simulink library "TYPEC_MASTER"  (Simulink 8.8)
settings: Solver=ode45  StartTime=0.0  StopTime=10.0  RelTol=1e-3  EnableMultiTasking=on
libraries: cdsEpicsOut x60, cdsFilt x45, cdsTP x20, cdsEpicsIn x18, cdsFiltCtrl x18, VIS_LIB x16, cdsMuxMatrix x8, cdsEpicsStringIn x6, cdsEpicsBinIn x4, lockin x4, cdsFunctionCall x4, STATE_BIO_MASTER x2
(part 1 of 7)
settings Model: SuppressorTable=22 serialization::archive 11 0 3 0 0 0 11 0  Creator=controls  LastModifiedBy=controls

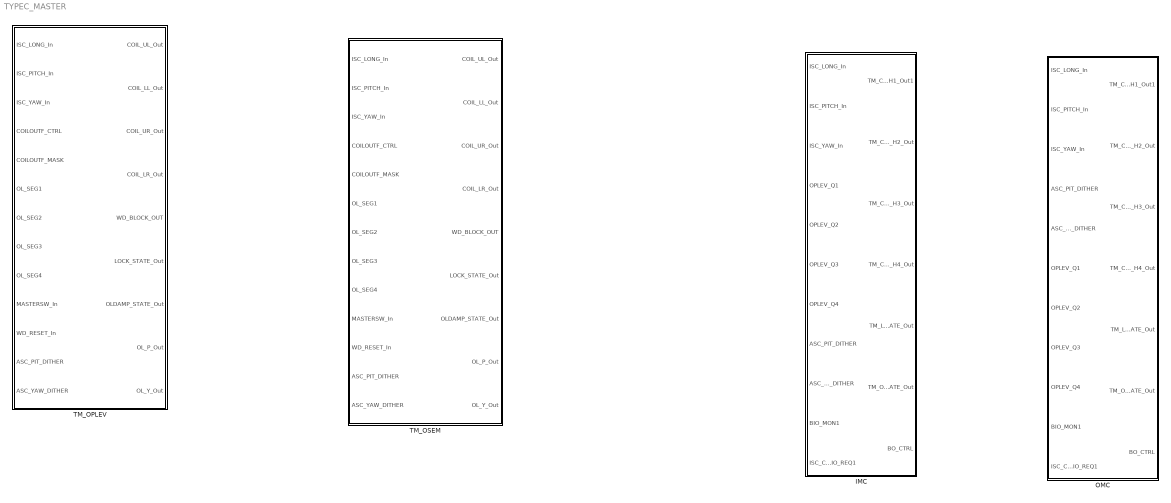
== system TYPEC_MASTER ==
  IMC : Subsystem  Description=TYPEC SINGLE MASTER
      settings: AttributesFormatString=%<Description>
  OMC : Subsystem  Description=TYPEC SINGLE MASTER
      settings: AttributesFormatString=%<Description>
  TM_OPLEV : Subsystem
  TM_OSEM : Subsystem

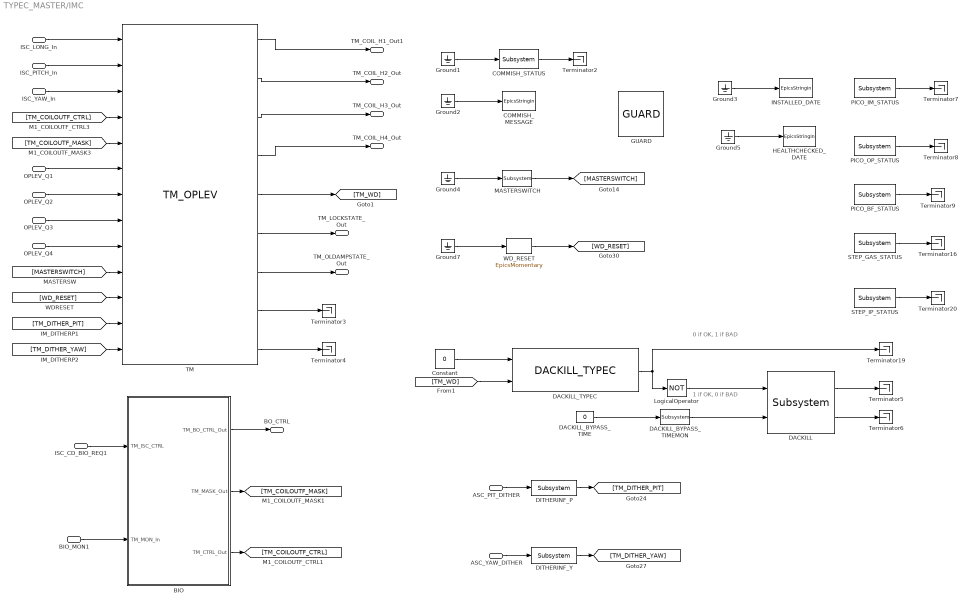
== system TYPEC_MASTER/IMC ==
  note: 0 if OK, 1 if BAD
  note: 1 if OK, 0 if BAD
  ISC_LONG_In : Inport
  ISC_PITCH_In : Inport  Port=2
  ISC_YAW_In : Inport  Port=3
  OPLEV_Q1 : Inport  Port=4
  OPLEV_Q2 : Inport  Port=5
  OPLEV_Q3 : Inport  Port=6
  OPLEV_Q4 : Inport  Port=7
  ASC_PIT_DITHER : Inport  Port=8
  ASC_YAW_DITHER : Inport  Port=9
  BIO_MON1 : Inport  Port=10
  ISC_CD_BIO_REQ1 : Inport  Port=11
  BIO : Subsystem
  COMMISH_MESSAGE : cdsEpicsStringIn/EpicsStringIn  Tag=cdsEpicsStringIn  Description=cdsEpicsStringIn
      settings: AttributesFormatString=%<Tag>
  COMMISH_STATUS : cdsEpicsBinIn/Subsystem  Tag=cdsEpicsBinIn  Description=|
      | Purpose:                                                                            
      | Create an EPICS binary (0 or 1) input channel to the FE realtime controls.          
      |                                                                                     
      | Operation:                                                                          
      | Outputs value from an EPICS ai record. Value is binary input (bi Epics record type).
      |                                                                                     
      | Usage:                                                                              
      | Name the part with the desired EPICS channel name.
      settings: AttributesFormatString=%<Tag>
  Constant : Constant  Value=0
  DACKILL : cdsDacKill/Subsystem  Description=cdsDacKill
      settings: AttributesFormatString=%<Description>
  DACKILL_BYPASS_TIME : Constant  Value=0
  DACKILL_BYPASS_TIMEMON : cdsEpicsOut/Subsystem  Tag=cdsEpicsOutput  Description=|
      | Purpose:                                          
      | Output a FE signal to an EPICS channel.           
      |                                                   
      | Operation:                                        
      | Takes input value and passes it to EPICS record.  
      |                                                   
      | Usage:                                            
      | Name the part with the desired EPICS rrecord name.
      settings: AttributesFormatString=%<Tag>
  DACKILL_TYPEC : VIS_LIB/DACKILL_TYPEC 
  DITHERINF_P : cdsFilt/Subsystem  Tag=cdsFilt  Description=|
      | Purpose:                                                                                                                                                                                                                                  
      | Standard CDS IIR filter module.                                                                                                                                                                                                           
      |                                                                                                                                                                                                                                           
      | Operation:                                                                                                                                                                                                                                
      | Consists of 10 second order section IIR filters, plus a ramped gain stage. In FE code, also provides pre-defined test points and excitation channel inputs. The filter coefficients are defined in the LIGO system using the 'foton' tool.
      |                                                                                                                                                                                                                                           
      | Usage:                                                                                                                                                                                                                                    
      | Name the part with the desired filter module name.
      settings: AttributesFormatString=%<Tag>
  DITHERINF_Y : cdsFilt/Subsystem  Tag=cdsFilt  Description=|
      | Purpose:                                                                                                                                                                                                                                  
      | Standard CDS IIR filter module.                                                                                                                                                                                                           
      |                                                                                                                                                                                                                                           
      | Operation:                                                                                                                                                                                                                                
      | Consists of 10 second order section IIR filters, plus a ramped gain stage. In FE code, also provides pre-defined test points and excitation channel inputs. The filter coefficients are defined in the LIGO system using the 'foton' tool.
      |                                                                                                                                                                                                                                           
      | Usage:                                                                                                                                                                                                                                    
      | Name the part with the desired filter module name.
      settings: AttributesFormatString=%<Tag>
  GUARD : ISC_common/GUARD
  Ground{1..5,7} (6 alike) : Ground
  HEALTHCHECKED_DATE : cdsEpicsStringIn/EpicsStringIn  Tag=cdsEpicsStringIn  Description=cdsEpicsStringIn
      settings: AttributesFormatString=%<Tag>
  INSTALLED_DATE : cdsEpicsStringIn/EpicsStringIn  Tag=cdsEpicsStringIn  Description=cdsEpicsStringIn
      settings: AttributesFormatString=%<Tag>
  LogicalOperator : Logic  Operator=NOT  AllPortsSameDT=off  OutDataTypeStr=boolean
  MASTERSWITCH : cdsEpicsBinIn/Subsystem  Tag=cdsEpicsBinIn  Description=|
      | Purpose:                                                                            
      | Create an EPICS binary (0 or 1) input channel to the FE realtime controls.          
      |                                                                                     
      | Operation:                                                                          
      | Outputs value from an EPICS ai record. Value is binary input (bi Epics record type).
      |                                                                                     
      | Usage:                                                                              
      | Name the part with the desired EPICS channel name.
      settings: AttributesFormatString=%<Tag>
  PICO_BF_STATUS : cdsEpicsIn/Subsystem  Tag=cdsEpicsIn  Description=|
      | Purpose:                                                                              
      | Create an EPICS input channel connection to the FE realtime controls.                 
      |                                                                                       
      | Operation:                                                                            
      | Outputs value from an EPICS ai record. Value is floating point with a precision of 3..
      |                                                                                       
      | Usage:                                                                                
      | Name the part with the desired EPICS channel name.
      settings: AttributesFormatString=%<Tag>
  PICO_IM_STATUS : cdsEpicsIn/Subsystem  Tag=cdsEpicsIn  Description=|
      | Purpose:                                                                              
      | Create an EPICS input channel connection to the FE realtime controls.                 
      |                                                                                       
      | Operation:                                                                            
      | Outputs value from an EPICS ai record. Value is floating point with a precision of 3..
      |                                                                                       
      | Usage:                                                                                
      | Name the part with the desired EPICS channel name.
      settings: AttributesFormatString=%<Tag>
  PICO_OP_STATUS : cdsEpicsIn/Subsystem  Tag=cdsEpicsIn  Description=|
      | Purpose:                                                                              
      | Create an EPICS input channel connection to the FE realtime controls.                 
      |                                                                                       
      | Operation:                                                                            
      | Outputs value from an EPICS ai record. Value is floating point with a precision of 3..
      |                                                                                       
      | Usage:                                                                                
      | Name the part with the desired EPICS channel name.
      settings: AttributesFormatString=%<Tag>
  STEP_GAS_STATUS : cdsEpicsIn/Subsystem  Tag=cdsEpicsIn  Description=|
      | Purpose:                                                                              
      | Create an EPICS input channel connection to the FE realtime controls.                 
      |                                                                                       
      | Operation:                                                                            
      | Outputs value from an EPICS ai record. Value is floating point with a precision of 3..
      |                                                                                       
      | Usage:                                                                                
      | Name the part with the desired EPICS channel name.
      settings: AttributesFormatString=%<Tag>
  STEP_IP_STATUS : cdsEpicsIn/Subsystem  Tag=cdsEpicsIn  Description=|
      | Purpose:                                                                              
      | Create an EPICS input channel connection to the FE realtime controls.                 
      |                                                                                       
      | Operation:                                                                            
      | Outputs value from an EPICS ai record. Value is floating point with a precision of 3..
      |                                                                                       
      | Usage:                                                                                
      | Name the part with the desired EPICS channel name.
      settings: AttributesFormatString=%<Tag>
  TM : TYPEC_MASTER/TM_OPLEV
  Terminator{2..9,16,19..20} (11 alike) : Terminator
  WD_RESET : cdsEpicsMomentary/EpicsMomentary  Tag=cdsEpicsMomentary
      settings: AttributesFormatString=%<Tag>
  TM_COIL_H1_Out1 : Outport
  TM_COIL_H2_Out : Outport  Port=2
  TM_COIL_H3_Out : Outport  Port=3
  TM_COIL_H4_Out : Outport  Port=4
  TM_LOCKSTATE_Out : Outport  Port=5
  TM_OLDAMPSTATE_Out : Outport  Port=6
  BO_CTRL : Outport  Port=7
  wires:
  TM/9 -> Terminator4/1
  TM/2 -> TM_COIL_H2_Out/1
  TM/1 -> TM_COIL_H1_Out1/1
  TM/4 -> TM_COIL_H4_Out/1
  TM/3 -> TM_COIL_H3_Out/1
  [TM_WD] -> DACKILL_TYPEC/2
  Constant/1 -> DACKILL_TYPEC/1
  DACKILL_TYPEC/1 -> Terminator19/1, LogicalOperator/1
  LogicalOperator/1 -> DACKILL/1
  DACKILL_BYPASS_TIMEMON/1 -> DACKILL/2
  DACKILL_BYPASS_TIME/1 -> DACKILL_BYPASS_TIMEMON/1
  DACKILL/1 -> Terminator5/1
  DACKILL/2 -> Terminator6/1
  [TM_DITHER_YAW] -> TM/13
  [TM_DITHER_PIT] -> TM/12
  DITHERINF_Y/1 -> [TM_DITHER_YAW]
  DITHERINF_P/1 -> [TM_DITHER_PIT]
  ASC_PIT_DITHER/1 -> DITHERINF_P/1
  ASC_YAW_DITHER/1 -> DITHERINF_Y/1
  Ground1/1 -> COMMISH_STATUS/1
  COMMISH_STATUS/1 -> Terminator2/1
  Ground2/1 -> COMMISH_MESSAGE/1
  ISC_LONG_In/1 -> TM/1
  TM/5 -> [TM_WD]
  MASTERSWITCH/1 -> [MASTERSWITCH]
  Ground4/1 -> MASTERSWITCH/1
  OPLEV_Q1/1 -> TM/6
  OPLEV_Q2/1 -> TM/7
  OPLEV_Q3/1 -> TM/8
  ISC_PITCH_In/1 -> TM/2
  ISC_YAW_In/1 -> TM/3
  OPLEV_Q4/1 -> TM/9
  [MASTERSWITCH] -> TM/10
  Ground7/1 -> WD_RESET/1
  WD_RESET/1 -> [WD_RESET]
  [WD_RESET] -> TM/11
  BIO_MON1/1 -> BIO/2(TM_MON_In)
  ISC_CD_BIO_REQ1/1 -> BIO/1(TM_ISC_CTRL)
  BIO/2(TM_MASK_Out) -> [TM_COILOUTF_MASK]
  BIO/3(TM_CTRL_Out) -> [TM_COILOUTF_CTRL]
  [TM_COILOUTF_CTRL] -> TM/4
  [TM_COILOUTF_MASK] -> TM/5
  BIO/1(TM_BO_CTRL_Out) -> BO_CTRL/1
  TM/6 -> TM_LOCKSTATE_Out/1
  TM/7 -> TM_OLDAMPSTATE_Out/1
  TM/8 -> Terminator3/1
  Ground3/1 -> INSTALLED_DATE/1
  Ground5/1 -> HEALTHCHECKED_DATE/1
  STEP_IP_STATUS/1 -> Terminator20/1
  STEP_GAS_STATUS/1 -> Terminator16/1
  PICO_BF_STATUS/1 -> Terminator9/1
  PICO_IM_STATUS/1 -> Terminator7/1
  PICO_OP_STATUS/1 -> Terminator8/1

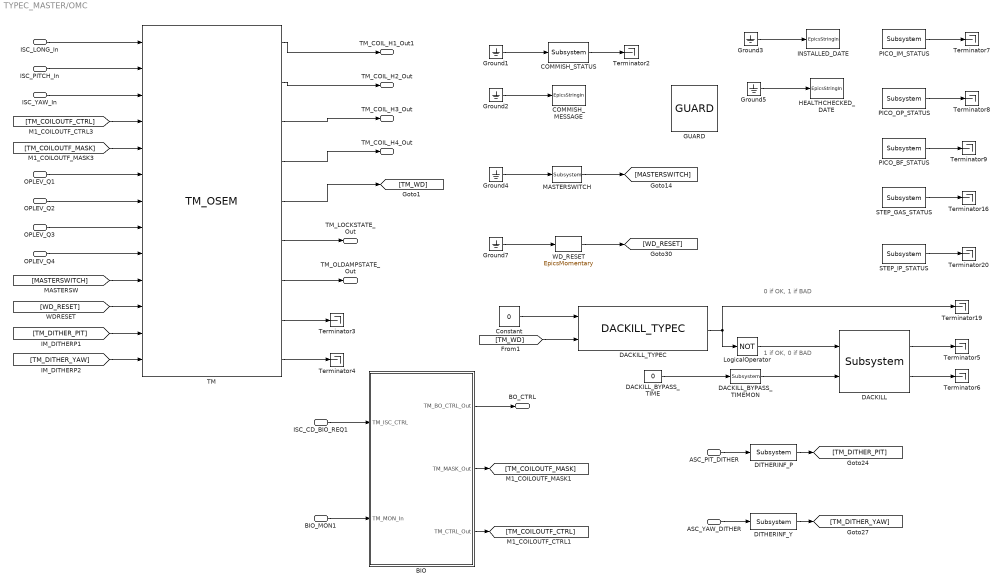
== system TYPEC_MASTER/OMC ==
  note: 0 if OK, 1 if BAD
  note: 1 if OK, 0 if BAD
  ISC_LONG_In : Inport
  ISC_PITCH_In : Inport  Port=2
  ISC_YAW_In : Inport  Port=3
  ASC_PIT_DITHER : Inport  Port=4
  ASC_YAW_DITHER : Inport  Port=5
  OPLEV_Q1 : Inport  Port=6
  OPLEV_Q2 : Inport  Port=7
  OPLEV_Q3 : Inport  Port=8
  OPLEV_Q4 : Inport  Port=9
  BIO_MON1 : Inport  Port=10
  ISC_CD_BIO_REQ1 : Inport  Port=11
  BIO : Subsystem
  COMMISH_MESSAGE : cdsEpicsStringIn/EpicsStringIn  Tag=cdsEpicsStringIn  Description=cdsEpicsStringIn
      settings: AttributesFormatString=%<Tag>
  COMMISH_STATUS : cdsEpicsBinIn/Subsystem  Tag=cdsEpicsBinIn  Description=|
      | Purpose:                                                                            
      | Create an EPICS binary (0 or 1) input channel to the FE realtime controls.          
      |                                                                                     
      | Operation:                                                                          
      | Outputs value from an EPICS ai record. Value is binary input (bi Epics record type).
      |                                                                                     
      | Usage:                                                                              
      | Name the part with the desired EPICS channel name.
      settings: AttributesFormatString=%<Tag>
  Constant : Constant  Value=0
  DACKILL : cdsDacKill/Subsystem  Description=cdsDacKill
      settings: AttributesFormatString=%<Description>
  DACKILL_BYPASS_TIME : Constant  Value=0
  DACKILL_BYPASS_TIMEMON : cdsEpicsOut/Subsystem  Tag=cdsEpicsOutput  Description=|
      | Purpose:                                          
      | Output a FE signal to an EPICS channel.           
      |                                                   
      | Operation:                                        
      | Takes input value and passes it to EPICS record.  
      |                                                   
      | Usage:                                            
      | Name the part with the desired EPICS rrecord name.
      settings: AttributesFormatString=%<Tag>
  DACKILL_TYPEC : VIS_LIB/DACKILL_TYPEC 
  DITHERINF_P : cdsFilt/Subsystem  Tag=cdsFilt  Description=|
      | Purpose:                                                                                                                                                                                                                                  
      | Standard CDS IIR filter module.                                                                                                                                                                                                           
      |                                                                                                                                                                                                                                           
      | Operation:                                                                                                                                                                                                                                
      | Consists of 10 second order section IIR filters, plus a ramped gain stage. In FE code, also provides pre-defined test points and excitation channel inputs. The filter coefficients are defined in the LIGO system using the 'foton' tool.
      |                                                                                                                                                                                                                                           
      | Usage:                                                                                                                                                                                                                                    
      | Name the part with the desired filter module name.
      settings: AttributesFormatString=%<Tag>
  DITHERINF_Y : cdsFilt/Subsystem  Tag=cdsFilt  Description=|
      | Purpose:                                                                                                                                                                                                                                  
      | Standard CDS IIR filter module.                                                                                                                                                                                                           
      |                                                                                                                                                                                                                                           
      | Operation:                                                                                                                                                                                                                                
      | Consists of 10 second order section IIR filters, plus a ramped gain stage. In FE code, also provides pre-defined test points and excitation channel inputs. The filter coefficients are defined in the LIGO system using the 'foton' tool.
      |                                                                                                                                                                                                                                           
      | Usage:                                                                                                                                                                                                                                    
      | Name the part with the desired filter module name.
      settings: AttributesFormatString=%<Tag>
  GUARD : ISC_common/GUARD
  Ground{1..5,7} (6 alike) : Ground
  HEALTHCHECKED_DATE : cdsEpicsStringIn/EpicsStringIn  Tag=cdsEpicsStringIn  Description=cdsEpicsStringIn
      settings: AttributesFormatString=%<Tag>
  INSTALLED_DATE : cdsEpicsStringIn/EpicsStringIn  Tag=cdsEpicsStringIn  Description=cdsEpicsStringIn
      settings: AttributesFormatString=%<Tag>
  LogicalOperator : Logic  Operator=NOT  AllPortsSameDT=off  OutDataTypeStr=boolean
  MASTERSWITCH : cdsEpicsBinIn/Subsystem  Tag=cdsEpicsBinIn  Description=|
      | Purpose:                                                                            
      | Create an EPICS binary (0 or 1) input channel to the FE realtime controls.          
      |                                                                                     
      | Operation:                                                                          
      | Outputs value from an EPICS ai record. Value is binary input (bi Epics record type).
      |                                                                                     
      | Usage:                                                                              
      | Name the part with the desired EPICS channel name.
      settings: AttributesFormatString=%<Tag>
  PICO_BF_STATUS : cdsEpicsIn/Subsystem  Tag=cdsEpicsIn  Description=|
      | Purpose:                                                                              
      | Create an EPICS input channel connection to the FE realtime controls.                 
      |                                                                                       
      | Operation:                                                                            
      | Outputs value from an EPICS ai record. Value is floating point with a precision of 3..
      |                                                                                       
      | Usage:                                                                                
      | Name the part with the desired EPICS channel name.
      settings: AttributesFormatString=%<Tag>
  PICO_IM_STATUS : cdsEpicsIn/Subsystem  Tag=cdsEpicsIn  Description=|
      | Purpose:                                                                              
      | Create an EPICS input channel connection to the FE realtime controls.                 
      |                                                                                       
      | Operation:                                                                            
      | Outputs value from an EPICS ai record. Value is floating point with a precision of 3..
      |                                                                                       
      | Usage:                                                                                
      | Name the part with the desired EPICS channel name.
      settings: AttributesFormatString=%<Tag>
  PICO_OP_STATUS : cdsEpicsIn/Subsystem  Tag=cdsEpicsIn  Description=|
      | Purpose:                                                                              
      | Create an EPICS input channel connection to the FE realtime controls.                 
      |                                                                                       
      | Operation:                                                                            
      | Outputs value from an EPICS ai record. Value is floating point with a precision of 3..
      |                                                                                       
      | Usage:                                                                                
      | Name the part with the desired EPICS channel name.
      settings: AttributesFormatString=%<Tag>
  STEP_GAS_STATUS : cdsEpicsIn/Subsystem  Tag=cdsEpicsIn  Description=|
      | Purpose:                                                                              
      | Create an EPICS input channel connection to the FE realtime controls.                 
      |                                                                                       
      | Operation:                                                                            
      | Outputs value from an EPICS ai record. Value is floating point with a precision of 3..
      |                                                                                       
      | Usage:                                                                                
      | Name the part with the desired EPICS channel name.
      settings: AttributesFormatString=%<Tag>
  STEP_IP_STATUS : cdsEpicsIn/Subsystem  Tag=cdsEpicsIn  Description=|
      | Purpose:                                                                              
      | Create an EPICS input channel connection to the FE realtime controls.                 
      |                                                                                       
      | Operation:                                                                            
      | Outputs value from an EPICS ai record. Value is floating point with a precision of 3..
      |                                                                                       
      | Usage:                                                                                
      | Name the part with the desired EPICS channel name.
      settings: AttributesFormatString=%<Tag>
  TM : TYPEC_MASTER/TM_OSEM
  Terminator{2..9,16,19..20} (11 alike) : Terminator
  WD_RESET : cdsEpicsMomentary/EpicsMomentary  Tag=cdsEpicsMomentary
      settings: AttributesFormatString=%<Tag>
  TM_COIL_H1_Out1 : Outport
  TM_COIL_H2_Out : Outport  Port=2
  TM_COIL_H3_Out : Outport  Port=3
  TM_COIL_H4_Out : Outport  Port=4
  TM_LOCKSTATE_Out : Outport  Port=5
  TM_OLDAMPSTATE_Out : Outport  Port=6
  BO_CTRL : Outport  Port=7
  wires:
  TM/9 -> Terminator4/1
  TM/2 -> TM_COIL_H2_Out/1
  TM/1 -> TM_COIL_H1_Out1/1
  TM/4 -> TM_COIL_H4_Out/1
  TM/3 -> TM_COIL_H3_Out/1
  [TM_WD] -> DACKILL_TYPEC/2
  Constant/1 -> DACKILL_TYPEC/1
  DACKILL_TYPEC/1 -> Terminator19/1, LogicalOperator/1
  LogicalOperator/1 -> DACKILL/1
  DACKILL_BYPASS_TIMEMON/1 -> DACKILL/2
  DACKILL_BYPASS_TIME/1 -> DACKILL_BYPASS_TIMEMON/1
  DACKILL/1 -> Terminator5/1
  DACKILL/2 -> Terminator6/1
  [TM_DITHER_YAW] -> TM/13
  [TM_DITHER_PIT] -> TM/12
  DITHERINF_Y/1 -> [TM_DITHER_YAW]
  DITHERINF_P/1 -> [TM_DITHER_PIT]
  ASC_PIT_DITHER/1 -> DITHERINF_P/1
  ASC_YAW_DITHER/1 -> DITHERINF_Y/1
  Ground1/1 -> COMMISH_STATUS/1
  COMMISH_STATUS/1 -> Terminator2/1
  Ground2/1 -> COMMISH_MESSAGE/1
  ISC_LONG_In/1 -> TM/1
  TM/5 -> [TM_WD]
  MASTERSWITCH/1 -> [MASTERSWITCH]
  Ground4/1 -> MASTERSWITCH/1
  OPLEV_Q1/1 -> TM/6
  OPLEV_Q2/1 -> TM/7
  OPLEV_Q3/1 -> TM/8
  ISC_PITCH_In/1 -> TM/2
  ISC_YAW_In/1 -> TM/3
  OPLEV_Q4/1 -> TM/9
  [MASTERSWITCH] -> TM/10
  Ground7/1 -> WD_RESET/1
  WD_RESET/1 -> [WD_RESET]
  [WD_RESET] -> TM/11
  BIO_MON1/1 -> BIO/2(TM_MON_In)
  ISC_CD_BIO_REQ1/1 -> BIO/1(TM_ISC_CTRL)
  BIO/2(TM_MASK_Out) -> [TM_COILOUTF_MASK]
  BIO/3(TM_CTRL_Out) -> [TM_COILOUTF_CTRL]
  [TM_COILOUTF_CTRL] -> TM/4
  [TM_COILOUTF_MASK] -> TM/5
  BIO/1(TM_BO_CTRL_Out) -> BO_CTRL/1
  TM/6 -> TM_LOCKSTATE_Out/1
  TM/7 -> TM_OLDAMPSTATE_Out/1
  TM/8 -> Terminator3/1
  Ground3/1 -> INSTALLED_DATE/1
  Ground5/1 -> HEALTHCHECKED_DATE/1
  STEP_IP_STATUS/1 -> Terminator20/1
  STEP_GAS_STATUS/1 -> Terminator16/1
  PICO_BF_STATUS/1 -> Terminator9/1
  PICO_IM_STATUS/1 -> Terminator7/1
  PICO_OP_STATUS/1 -> Terminator8/1

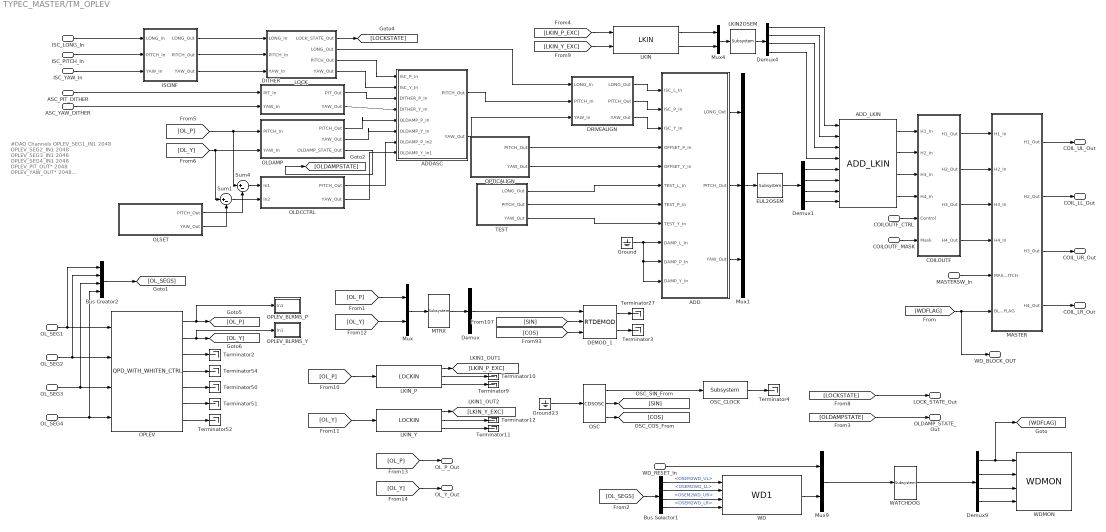
== system TYPEC_MASTER/TM_OPLEV ==
  note: #DAQ Channels
      | OPLEV_SEG1_IN1 2048
      | OPLEV_SEG2_IN1 2048
      | OPLEV_SEG3_IN1 2048
      | OPLEV_SEG4_IN1 2048
      | OPLEV_PIT_OUT* 2048
      | OPLEV_YAW_OUT* 2048
      | OPLEV_SUM_OUT 2048
      | ISCINF_L_IN1 2048
  ISC_LONG_In : Inport
  ISC_PITCH_In : Inport  Port=2
  ISC_YAW_In : Inport  Port=3
  COILOUTF_CTRL : Inport  Port=4
  COILOUTF_MASK : Inport  Port=5
  OL_SEG1 : Inport  Port=6
  OL_SEG2 : Inport  Port=7
  OL_SEG3 : Inport  Port=8
  OL_SEG4 : Inport  Port=9
  MASTERSW_In : Inport  Port=10
  WD_RESET_In : Inport  Port=11
  ASC_PIT_DITHER : Inport  Port=12
  ASC_YAW_DITHER : Inport  Port=13
  ADD : Subsystem
  ADDASC : Subsystem
  ADD_LKIN : VIS_LIB/ADD_LKIN
  Bus Creator2 : BusCreator  Inputs='OSEM2WD_UL','OSEM2WD_LL','OSEM2WD_UR','OSEM2WD_LR'
  Bus Selector1 : BusSelector  OutputSignals=OSEM2WD_UL,OSEM2WD_LL,OSEM2WD_UR,OSEM2WD_LR
  COILOUTF : Subsystem
  DEMOD_1 : VIS_LIB/RTDEMOD
  DITHER : Subsystem
  DRIVEALIGN : Subsystem
  Demux : Demux  Outputs=1
  Demux1 : Demux
  Demux4 : Demux
  Demux9 : Demux
  EUL2OSEM : cdsMuxMatrix/Subsystem  Tag=cdsMuxMatrix  Description=Any size matrix. Inputs and outputs must be connected using Mux and Demux parts.
      settings: AttributesFormatString=%<Tag>
  Ground : Ground
  Ground23 : Ground
  ISCINF : Subsystem
  LKIN : VIS_LIB/LKIN
  LKIN2OSEM : cdsMuxMatrix/Subsystem  Tag=cdsMuxMatrix  Description=Any size matrix. Inputs and outputs must be connected using Mux and Demux parts.
      settings: AttributesFormatString=%<Tag>
  LKIN_P : lockin/LOCKIN  Description=ADL=LOCKIN.adl
      settings: AttributesFormatString=%<Tag>
  LKIN_Y : lockin/LOCKIN  Description=ADL=LOCKIN.adl
      settings: AttributesFormatString=%<Tag>
  LOCK : Subsystem
  MASTER : Subsystem
  MTRX : cdsMuxMatrix/Subsystem  Tag=cdsMuxMatrix  Description=Any size matrix. Inputs and outputs must be connected using Mux and Demux parts.
      settings: AttributesFormatString=%<Tag>
  Mux : Mux  Inputs=2
  Mux1 : Mux  Inputs=3
  Mux4 : Mux  Inputs=2
  Mux9 : Mux  Inputs=2
  OLDAMP : Subsystem
  OLDCCTRL : Subsystem
  OLSET : Subsystem
  OPLEV : VIS_LIB/QPD_WITH_WHITEN_CTRL
  OPLEV_BLRMS_P : Subsystem
  OPLEV_BLRMS_Y : Subsystem
  OPTICALIGN : Subsystem
  OSC : VIS_LIB/CDSOSC  Description=ADL=OSC.adl
  OSC_CLOCK : cdsEpicsOut/Subsystem  Tag=cdsEpicsOutput  Description=|
      | Purpose:                                          
      | Output a FE signal to an EPICS channel.           
      |                                                   
      | Operation:                                        
      | Takes input value and passes it to EPICS record.  
      |                                                   
      | Usage:                                            
      | Name the part with the desired EPICS rrecord name.
      settings: AttributesFormatString=%<Tag>
  Sum1 : Sum  Inputs=|+-
  Sum4 : Sum  Inputs=|+-
  TEST : Subsystem
  Terminator{2..4,9..12,27,50..52,54} (12 alike) : Terminator
  WATCHDOG : cdsFunctionCall/Subsystem  Tag=cdsFunctionCall  Description=inline OSEMWATCHDOG /opt/rtcds/userapps/release/vis/common/src/WATCHDOG.c
      settings: AttributesFormatString=%<Tag>\n%<Description>
  WD : VIS_LIB/WD1
  WDMON : VIS_LIB/WDMON
  COIL_UL_Out : Outport
  COIL_LL_Out : Outport  Port=2
  COIL_UR_Out : Outport  Port=3
  COIL_LR_Out : Outport  Port=4
  WD_BLOCK_OUT : Outport  Port=5
  LOCK_STATE_Out : Outport  Port=6
  OLDAMP_STATE_Out : Outport  Port=7
  OL_P_Out : Outport  Port=8
  OL_Y_Out : Outport  Port=9
  wires:
  OLDCCTRL/2(YAW_Out) -> ADDASC/8(OLDAMP_Y_In1)
  OLDCCTRL/1(PITCH_Out) -> ADDASC/7(OLDAMP_P_In2)
  OLSET/2(YAW_Out) -> Sum1/2
  Sum1/1 -> OLDCCTRL/2(In2)
  Sum4/1 -> OLDCCTRL/1(In1)
  OLSET/1(PITCH_Out) -> Sum4/2
  MASTERSW_In/1 -> MASTER/5(MASTERSWITCH)
  COILOUTF/2(H2_Out) -> MASTER/2(H2_In)
  Ground/1 -> ADD/9(DAMP_L_In), ADD/11(DAMP_Y_In), ADD/10(DAMP_P_In)
  Bus Creator2/1 -> [OL_SEGS]
  [OL_Y] -> OL_Y_Out/1
  [OL_P] -> OL_P_Out/1
  [OL_Y] -> Mux/2
  [OL_P] -> Mux/1
  OSC/3 -> [COS]
  OSC/2 -> [SIN]
  OSC_CLOCK/1 -> Terminator4/1
  OSC/1 -> OSC_CLOCK/1
  Ground23/1 -> OSC/1
  DEMOD_1/2 -> Terminator3/1
  DEMOD_1/1 -> Terminator27/1
  [COS] -> DEMOD_1/3
  [SIN] -> DEMOD_1/2
  Demux/1 -> DEMOD_1/1
  MTRX/1 -> Demux/1
  Mux/1 -> MTRX/1
  ISCINF/3(YAW_Out) -> LOCK/3(YAW_In)
  ISCINF/2(PITCH_Out) -> LOCK/2(PITCH_In)
  ISCINF/1(LONG_Out) -> LOCK/1(LONG_In)
  ISC_PITCH_In/1 -> ISCINF/2(PITCH_In)
  ISC_LONG_In/1 -> ISCINF/1(LONG_In)
  ISC_YAW_In/1 -> ISCINF/3(YAW_In)
  WD/1 -> Mux9/2
  [LKIN_Y_EXC] -> LKIN/2
  [LKIN_P_EXC] -> LKIN/1
  LKIN_Y/3 -> Terminator11/1
  LKIN_Y/2 -> Terminator12/1
  [OL_Y] -> LKIN_Y/1
  LKIN_Y/1 -> [LKIN_Y_EXC]
  LKIN_P/1 -> [LKIN_P_EXC]
  LKIN_P/3 -> Terminator9/1
  LKIN_P/2 -> Terminator10/1
  [OL_P] -> LKIN_P/1
  LOCK/1(LOCK_STATE_Out) -> [LOCKSTATE]
  [OLDAMPSTATE] -> OLDAMP_STATE_Out/1
  [LOCKSTATE] -> LOCK_STATE_Out/1
  ADD_LKIN/4 -> COILOUTF/4(H4_In)
  ADD_LKIN/3 -> COILOUTF/3(H3_In)
  ADD_LKIN/2 -> COILOUTF/2(H2_In)
  ADD_LKIN/1 -> COILOUTF/1(H1_In)
  Demux1/4 -> ADD_LKIN/8
  Demux1/3 -> ADD_LKIN/7
  Demux1/2 -> ADD_LKIN/6
  Demux1/1 -> ADD_LKIN/5
  Demux4/4 -> ADD_LKIN/4
  Demux4/3 -> ADD_LKIN/3
  Demux4/2 -> ADD_LKIN/2
  LKIN/2 -> Mux4/2
  LKIN/1 -> Mux4/1
  Demux4/1 -> ADD_LKIN/1
  LKIN2OSEM/1 -> Demux4/1
  Mux4/1 -> LKIN2OSEM/1
  MASTER/4(H4_Out) -> COIL_LR_Out/1
  MASTER/3(H3_Out) -> COIL_UR_Out/1
  MASTER/2(H2_Out) -> COIL_LL_Out/1
  MASTER/1(H1_Out) -> COIL_UL_Out/1
  OPLEV/7 -> Terminator52/1
  OPLEV/6 -> Terminator51/1
  OPLEV/5 -> Terminator50/1
  OPLEV/4 -> Terminator54/1
  OLDAMP/3(OLDAMP_STATE_Out) -> [OLDAMPSTATE]
  OPLEV/3 -> Terminator2/1
  OPLEV/1 -> [OL_P], OPLEV_BLRMS_P/1(In1)
  OPLEV/2 -> [OL_Y], OPLEV_BLRMS_Y/1(In1)
  DRIVEALIGN/3(YAW_Out) -> ADD/3(ISC_Y_In)
  DRIVEALIGN/2(PITCH_Out) -> ADD/2(ISC_P_In)
  DRIVEALIGN/1(LONG_Out) -> ADD/1(ISC_L_In)
  ADDASC/2(YAW_Out) -> DRIVEALIGN/3(YAW_In)
  ADDASC/1(PITCH_Out) -> DRIVEALIGN/2(PITCH_In)
  LOCK/2(LONG_Out) -> DRIVEALIGN/1(LONG_In)
  ADD/1(LONG_Out) -> Mux1/1
  ADD/2(PITCH_Out) -> Mux1/2
  ADD/3(YAW_Out) -> Mux1/3
  OLDAMP/2(YAW_Out) -> ADDASC/6(OLDAMP_Y_In)
  OLDAMP/1(PITCH_Out) -> ADDASC/5(OLDAMP_P_In)
  DITHER/2(YAW_Out) -> ADDASC/4(DITHER_Y_In)
  DITHER/1(PIT_Out) -> ADDASC/3(DITHER_P_In)
  LOCK/4(YAW_Out) -> ADDASC/2(ISC_Y_In)
  [OL_Y] -> OLDAMP/2(YAW_In), Sum1/1
  [OL_P] -> OLDAMP/1(PITCH_In), Sum4/1
  ASC_YAW_DITHER/1 -> DITHER/2(YAW_In)
  ASC_PIT_DITHER/1 -> DITHER/1(PIT_In)
  OL_SEG4/1 -> OPLEV/4, Bus Creator2/4
  OL_SEG3/1 -> OPLEV/3, Bus Creator2/3
  OL_SEG2/1 -> OPLEV/2, Bus Creator2/2
  OL_SEG1/1 -> OPLEV/1, Bus Creator2/1
  Bus Selector1/4 -> WD/4  "<OSEM2WD_LR>"
  Bus Selector1/3 -> WD/3  "<OSEM2WD_UR>"
  Bus Selector1/2 -> WD/2  "<OSEM2WD_LL>"
  Bus Selector1/1 -> WD/1  "<OSEM2WD_UL>"
  [OL_SEGS] -> Bus Selector1/1
  Mux1/1 -> EUL2OSEM/1
  EUL2OSEM/1 -> Demux1/1
  Demux9/1 -> [WDFLAG], WDMON/1
  Demux9/2 -> WDMON/2
  Demux9/3 -> WDMON/3
  Demux9/4 -> WDMON/4
  WATCHDOG/1 -> Demux9/1
  Mux9/1 -> WATCHDOG/1
  [WDFLAG] -> MASTER/6(BLOCKFLAG), WD_BLOCK_OUT/1
  COILOUTF/1(H1_Out) -> MASTER/1(H1_In)
  COILOUTF/3(H3_Out) -> MASTER/3(H3_In)
  COILOUTF/4(H4_Out) -> MASTER/4(H4_In)
  WD_RESET_In/1 -> Mux9/1
  COILOUTF_MASK/1 -> COILOUTF/6(Mask)
  COILOUTF_CTRL/1 -> COILOUTF/5(Control)
  TEST/1(LONG_Out) -> ADD/6(TEST_L_In)
  TEST/2(PITCH_Out) -> ADD/7(TEST_P_In)
  TEST/3(YAW_Out) -> ADD/8(TEST_Y_In)
  LOCK/3(PITCH_Out) -> ADDASC/1(ISC_P_In)
  OPTICALIGN/1(PITCH_Out) -> ADD/4(OFFSET_P_In)
  OPTICALIGN/2(YAW_Out) -> ADD/5(OFFSET_Y_In)

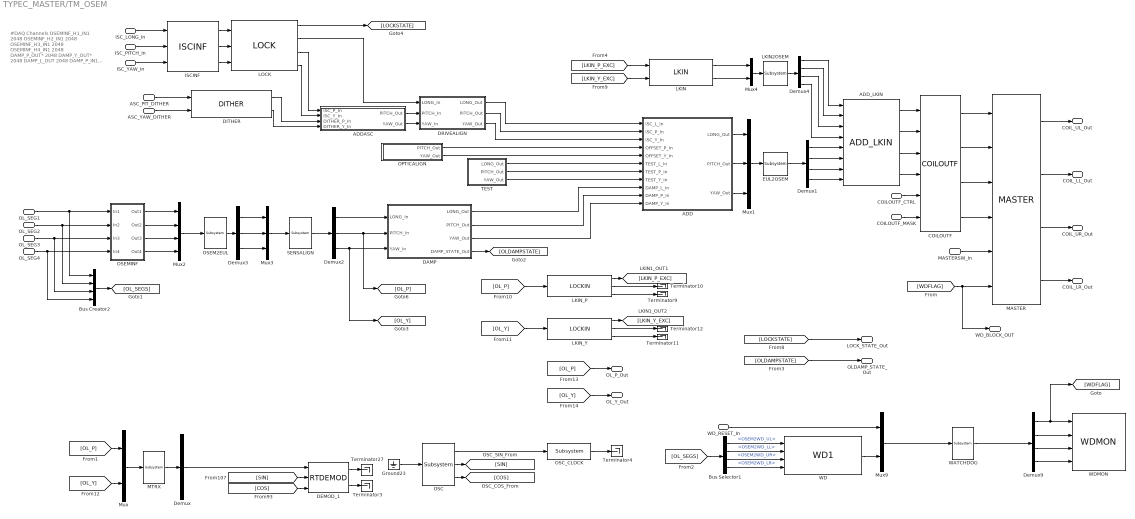
== system TYPEC_MASTER/TM_OSEM ==
  note: #DAQ Channels
      | OSEMINF_H1_IN1 2048
      | OSEMINF_H2_IN1 2048
      | OSEMINF_H3_IN1 2048
      | OSEMINF_H4_IN1 2048
      | DAMP_P_OUT* 2048
      | DAMP_Y_OUT* 2048
      | DAMP_L_OUT 2048
      | DAMP_P_IN1 2048
      | DAMP_Y_IN1 2048
      | DAMP_L_IN1 2048
      | ISCINF_L_IN1 2048
  ISC_LONG_In : Inport
  ISC_PITCH_In : Inport  Port=2
  ISC_YAW_In : Inport  Port=3
  COILOUTF_CTRL : Inport  Port=4
  COILOUTF_MASK : Inport  Port=5
  OL_SEG1 : Inport  Port=6
  OL_SEG2 : Inport  Port=7
  OL_SEG3 : Inport  Port=8
  OL_SEG4 : Inport  Port=9
  MASTERSW_In : Inport  Port=10
  WD_RESET_In : Inport  Port=11
  ASC_PIT_DITHER : Inport  Port=12
  ASC_YAW_DITHER : Inport  Port=13
  ADD : Subsystem
  ADDASC : Subsystem
  ADD_LKIN : VIS_LIB/ADD_LKIN
  Bus Creator2 : BusCreator  Inputs='OSEM2WD_UL','OSEM2WD_LL','OSEM2WD_UR','OSEM2WD_LR'
  Bus Selector1 : BusSelector  OutputSignals=OSEM2WD_UL,OSEM2WD_LL,OSEM2WD_UR,OSEM2WD_LR
  COILOUTF : FOUROSEM_COILOUTF_MASTER/COILOUTF
  DAMP : Subsystem
  DEMOD_1 : rtdemod/RTDEMOD  Tag=top_names
  DITHER : VIS_LIB/DITHER
  DRIVEALIGN : Subsystem
  Demux : Demux  Outputs=1
  Demux1 : Demux
  Demux2 : Demux  Outputs=3
  Demux3 : Demux  Outputs=3
  Demux4 : Demux
  Demux9 : Demux
  EUL2OSEM : cdsMuxMatrix/Subsystem  Tag=cdsMuxMatrix  Description=Any size matrix. Inputs and outputs must be connected using Mux and Demux parts.
      settings: AttributesFormatString=%<Tag>
  Ground23 : Ground
  ISCINF : VIS_LIB/ISCINF
  LKIN : VIS_LIB/LKIN
  LKIN2OSEM : cdsMuxMatrix/Subsystem  Tag=cdsMuxMatrix  Description=Any size matrix. Inputs and outputs must be connected using Mux and Demux parts.
      settings: AttributesFormatString=%<Tag>
  LKIN_P : lockin/LOCKIN  Description=ADL=LOCKIN.adl
      settings: AttributesFormatString=%<Tag>
  LKIN_Y : lockin/LOCKIN  Description=ADL=LOCKIN.adl
      settings: AttributesFormatString=%<Tag>
  LOCK : VIS_LIB/LOCK
  MASTER : CRYP_TM_MASTER/CRYP_TM_MASTER/MASTER
  MTRX : cdsMuxMatrix/Subsystem  Tag=cdsMuxMatrix  Description=Any size matrix. Inputs and outputs must be connected using Mux and Demux parts.
      settings: AttributesFormatString=%<Tag>
  Mux : Mux  Inputs=2
  Mux1 : Mux  Inputs=3
  Mux2 : Mux
  Mux3 : Mux  Inputs=3
  Mux4 : Mux  Inputs=2
  Mux9 : Mux  Inputs=2
  OPTICALIGN : Subsystem
  OSC : cdsOsc/Subsystem  Tag=cdsOsc  Description=Oscillator
      settings: AttributesFormatString=%<Tag>
  OSC_CLOCK : cdsEpicsOut/Subsystem  Tag=cdsEpicsOutput  Description=|
      | Purpose:                                          
      | Output a FE signal to an EPICS channel.           
      |                                                   
      | Operation:                                        
      | Takes input value and passes it to EPICS record.  
      |                                                   
      | Usage:                                            
      | Name the part with the desired EPICS rrecord name.
      settings: AttributesFormatString=%<Tag>
  OSEM2EUL : cdsMuxMatrix/Subsystem  Tag=cdsMuxMatrix  Description=Any size matrix. Inputs and outputs must be connected using Mux and Demux parts.
      settings: AttributesFormatString=%<Tag>
  OSEMINF : Subsystem
  SENSALIGN : cdsMuxMatrix/Subsystem  Tag=cdsMuxMatrix  Description=Any size matrix. Inputs and outputs must be connected using Mux and Demux parts.
      settings: AttributesFormatString=%<Tag>
  TEST : Subsystem
  Terminator{3..4,9..12,27} (7 alike) : Terminator
  WATCHDOG : cdsFunctionCall/Subsystem  Tag=cdsFunctionCall  Description=inline OSEMWATCHDOG /opt/rtcds/userapps/release/vis/common/src/WATCHDOG.c
      settings: AttributesFormatString=%<Tag>\n%<Description>
  WD : VIS_LIB/WD1
  WDMON : VIS_LIB/WDMON
  COIL_UL_Out : Outport
  COIL_LL_Out : Outport  Port=2
  COIL_UR_Out : Outport  Port=3
  COIL_LR_Out : Outport  Port=4
  WD_BLOCK_OUT : Outport  Port=5
  LOCK_STATE_Out : Outport  Port=6
  OLDAMP_STATE_Out : Outport  Port=7
  OL_P_Out : Outport  Port=8
  OL_Y_Out : Outport  Port=9
  wires:
  OSEMINF/4(Out4) -> Mux2/4
  OSEMINF/3(Out3) -> Mux2/3
  OSEMINF/2(Out2) -> Mux2/2
  OSEMINF/1(Out1) -> Mux2/1
  SENSALIGN/1 -> Demux2/1
  Demux3/3 -> Mux3/3
  Demux3/2 -> Mux3/2
  Demux3/1 -> Mux3/1
  OSEM2EUL/1 -> Demux3/1
  Mux3/1 -> SENSALIGN/1
  Demux2/3 -> DAMP/3(YAW_In), [OL_Y]
  Demux2/2 -> DAMP/2(PITCH_In), [OL_P]
  Demux2/1 -> DAMP/1(LONG_In)
  Mux2/1 -> OSEM2EUL/1
  ASC_PIT_DITHER/1 -> DITHER/1
  DAMP/3(YAW_Out) -> ADD/11(DAMP_Y_In)
  DAMP/2(PITCH_Out) -> ADD/10(DAMP_P_In)
  DAMP/1(LONG_Out) -> ADD/9(DAMP_L_In)
  DITHER/2 -> ADDASC/4(DITHER_Y_In)
  DAMP/4(DAMP_STATE_Out) -> [OLDAMPSTATE]
  OPTICALIGN/2(YAW_Out) -> ADD/5(OFFSET_Y_In)
  OPTICALIGN/1(PITCH_Out) -> ADD/4(OFFSET_P_In)
  LOCK/3 -> ADDASC/1(ISC_P_In)
  TEST/3(YAW_Out) -> ADD/8(TEST_Y_In)
  TEST/2(PITCH_Out) -> ADD/7(TEST_P_In)
  TEST/1(LONG_Out) -> ADD/6(TEST_L_In)
  COILOUTF_CTRL/1 -> COILOUTF/5
  COILOUTF_MASK/1 -> COILOUTF/6
  WD_RESET_In/1 -> Mux9/1
  COILOUTF/4 -> MASTER/4
  COILOUTF/3 -> MASTER/3
  COILOUTF/1 -> MASTER/1
  [WDFLAG] -> WD_BLOCK_OUT/1, MASTER/6
  Mux9/1 -> WATCHDOG/1
  WATCHDOG/1 -> Demux9/1
  Demux9/4 -> WDMON/4
  Demux9/3 -> WDMON/3
  Demux9/2 -> WDMON/2
  Demux9/1 -> WDMON/1, [WDFLAG]
  EUL2OSEM/1 -> Demux1/1
  Mux1/1 -> EUL2OSEM/1
  [OL_SEGS] -> Bus Selector1/1
  Bus Selector1/1 -> WD/1  "<OSEM2WD_UL>"
  Bus Selector1/2 -> WD/2  "<OSEM2WD_LL>"
  Bus Selector1/3 -> WD/3  "<OSEM2WD_UR>"
  Bus Selector1/4 -> WD/4  "<OSEM2WD_LR>"
  OL_SEG1/1 -> Bus Creator2/1, OSEMINF/1(In1)
  OL_SEG2/1 -> Bus Creator2/2, OSEMINF/2(In2)
  OL_SEG3/1 -> Bus Creator2/3, OSEMINF/3(In3)
  OL_SEG4/1 -> Bus Creator2/4, OSEMINF/4(In4)
  ASC_YAW_DITHER/1 -> DITHER/2
  LOCK/4 -> ADDASC/2(ISC_Y_In)
  DITHER/1 -> ADDASC/3(DITHER_P_In)
  ADD/3(YAW_Out) -> Mux1/3
  ADD/2(PITCH_Out) -> Mux1/2
  ADD/1(LONG_Out) -> Mux1/1
  LOCK/2 -> DRIVEALIGN/1(LONG_In)
  ADDASC/1(PITCH_Out) -> DRIVEALIGN/2(PITCH_In)
  ADDASC/2(YAW_Out) -> DRIVEALIGN/3(YAW_In)
  DRIVEALIGN/1(LONG_Out) -> ADD/1(ISC_L_In)
  DRIVEALIGN/2(PITCH_Out) -> ADD/2(ISC_P_In)
  DRIVEALIGN/3(YAW_Out) -> ADD/3(ISC_Y_In)
  MASTER/1 -> COIL_UL_Out/1
  MASTER/2 -> COIL_LL_Out/1
  MASTER/3 -> COIL_UR_Out/1
  MASTER/4 -> COIL_LR_Out/1
  Mux4/1 -> LKIN2OSEM/1
  LKIN2OSEM/1 -> Demux4/1
  Demux4/1 -> ADD_LKIN/1
  LKIN/1 -> Mux4/1
  LKIN/2 -> Mux4/2
  Demux4/2 -> ADD_LKIN/2
  Demux4/3 -> ADD_LKIN/3
  Demux4/4 -> ADD_LKIN/4
  Demux1/1 -> ADD_LKIN/5
  Demux1/2 -> ADD_LKIN/6
  Demux1/3 -> ADD_LKIN/7
  Demux1/4 -> ADD_LKIN/8
  ADD_LKIN/1 -> COILOUTF/1
  ADD_LKIN/2 -> COILOUTF/2
  ADD_LKIN/3 -> COILOUTF/3
  ADD_LKIN/4 -> COILOUTF/4
  [LOCKSTATE] -> LOCK_STATE_Out/1
  [OLDAMPSTATE] -> OLDAMP_STATE_Out/1
  LOCK/1 -> [LOCKSTATE]
  [OL_P] -> LKIN_P/1
  LKIN_P/2 -> Terminator10/1
  LKIN_P/3 -> Terminator9/1
  LKIN_P/1 -> [LKIN_P_EXC]
  LKIN_Y/1 -> [LKIN_Y_EXC]
  [OL_Y] -> LKIN_Y/1
  LKIN_Y/2 -> Terminator12/1
  LKIN_Y/3 -> Terminator11/1
  [LKIN_P_EXC] -> LKIN/1
  [LKIN_Y_EXC] -> LKIN/2
  WD/1 -> Mux9/2
  ISC_YAW_In/1 -> ISCINF/3
  ISC_LONG_In/1 -> ISCINF/1
  ISC_PITCH_In/1 -> ISCINF/2
  ISCINF/1 -> LOCK/1
  ISCINF/2 -> LOCK/2
  ISCINF/3 -> LOCK/3
  Mux/1 -> MTRX/1
  MTRX/1 -> Demux/1
  Demux/1 -> DEMOD_1/1
  [SIN] -> DEMOD_1/2
  [COS] -> DEMOD_1/3
  DEMOD_1/1 -> Terminator27/1
  DEMOD_1/2 -> Terminator3/1
  Ground23/1 -> OSC/1
  OSC/1 -> OSC_CLOCK/1
  OSC_CLOCK/1 -> Terminator4/1
  OSC/2 -> [SIN]
  OSC/3 -> [COS]
  [OL_P] -> Mux/1
  [OL_Y] -> Mux/2
  [OL_P] -> OL_P_Out/1
  [OL_Y] -> OL_Y_Out/1
  Bus Creator2/1 -> [OL_SEGS]
  COILOUTF/2 -> MASTER/2
  MASTERSW_In/1 -> MASTER/5

== system TYPEC_MASTER/IMC/BIO ==
  note: 12 Bit Word
  note: 12 Bit Word
  TM_ISC_CTRL : Inport
  TM_MON_In : Inport  Port=2
  TM : STATE_BIO_MASTER/UIM_BIO_MASTER
  TM_BO_CTRL_Out : Outport
  TM_MASK_Out : Outport  Port=2
  TM_CTRL_Out : Outport  Port=3
  wires:
  TM/2 -> TM_CTRL_Out/1
  TM/1 -> TM_MASK_Out/1
  TM/3 -> TM_BO_CTRL_Out/1
  TM_MON_In/1 -> TM/2
  TM_ISC_CTRL/1 -> TM/1

== system TYPEC_MASTER/OMC/BIO ==
  note: 12 Bit Word
  note: 12 Bit Word
  TM_ISC_CTRL : Inport
  TM_MON_In : Inport  Port=2
  TM : STATE_BIO_MASTER/UIM_BIO_MASTER
  TM_BO_CTRL_Out : Outport
  TM_MASK_Out : Outport  Port=2
  TM_CTRL_Out : Outport  Port=3
  wires:
  TM/2 -> TM_CTRL_Out/1
  TM/1 -> TM_MASK_Out/1
  TM/3 -> TM_BO_CTRL_Out/1
  TM_MON_In/1 -> TM/2
  TM_ISC_CTRL/1 -> TM/1
